simulink model "Model_01_work_2017"  (R2017a)
settings: Solver=VariableStepAuto  StartTime=0.0  StopTime=96  RelTol=1e-3
settings Model: Creator=alexandr.lanin  LastModifiedBy=alexandr.lanin

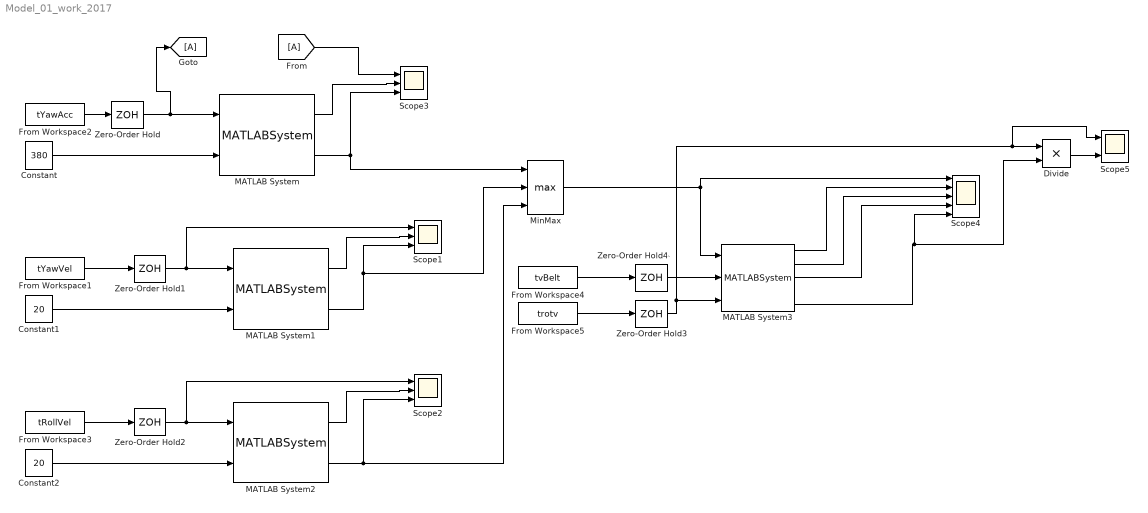
== system Model_01_work_2017 ==
  note: `
  Constant : Constant  Value=380
  Constant1 : Constant  Value=20
  Constant2 : Constant  Value=20
  Divide : Product  Inputs=**
  From Workspace1 : FromWorkspace  VariableName=tYawVel  SampleTime=0
  From Workspace2 : FromWorkspace  VariableName=tYawAcc  SampleTime=0
  From Workspace3 : FromWorkspace  VariableName=tRollVel  SampleTime=0
  From Workspace4 : FromWorkspace  VariableName=tvBelt  SampleTime=0
  From Workspace5 : FromWorkspace  VariableName=trotv  SampleTime=0
  MATLAB System : MATLABSystem  System=WolchSimCode  kMul=100  SimulateUsing=Code generation
      mask Type: WolchSimCode
      mask Display:
      | disp('WolchSimCode');
      | port_label('input',1,'u');
      | port_label('input',2,'norm');
      | port_label('output',1,'Y');
      | port_label('output',2,'Ynorm');
  MATLAB System1 : MATLABSystem  System=WolchSimCode  kMul=100  SimulateUsing=Code generation
      mask Type: WolchSimCode
      mask Display:
      | disp('WolchSimCode');
      | port_label('input',1,'u');
      | port_label('input',2,'norm');
      | port_label('output',1,'Y');
      | port_label('output',2,'Ynorm');
  MATLAB System2 : MATLABSystem  System=WolchSimCode  kMul=100  SimulateUsing=Code generation
      mask Type: WolchSimCode
      mask Display:
      | disp('WolchSimCode');
      | port_label('input',1,'u');
      | port_label('input',2,'norm');
      | port_label('output',1,'Y');
      | port_label('output',2,'Ynorm');
  MATLAB System3 : MATLABSystem  System=ModulSigmoid  Rwheel=17*0.0254  Transfer=3  Kreset=0.6  sd=6  sdsn=0.25  betta=0.6  sm_bet=0.3  alfa=1.0  sm_alfa=0.3  kStd=4  alfaExp=0.75  SimulateUsing=Code generation
      mask Type: ModulSigmoid
      mask Display:
      | disp('ModulSigmoid');
      | port_label('input',1,'signal');
      | port_label('input',2,'vBelt');
      | port_label('input',3,'rotv');
      | port_label('output',1,'y');
      | port_label('output',2,'k');
      | port_label('output',3,'v');
      | port_label('output',4,'ye');
      | port_label('output',5,'yinver');
  MinMax : MinMax  Function=max  Inputs=3
  Scope1 : Scope  NumInputPorts=3
  Scope2 : Scope  NumInputPorts=3
  Scope3 : Scope  NumInputPorts=3
  Scope4 : Scope  NumInputPorts=5
  Scope5 : Scope  NumInputPorts=2
  Zero-Order Hold{,1..4} (5 alike) : ZeroOrderHold  SampleTime=0.01
  wires:
  From Workspace2/1 -> Zero-Order Hold/1
  Zero-Order Hold/1 -> [A], MATLAB System/1
  MATLAB System/1 -> Scope3/2
  MATLAB System/2 -> MinMax/1, Scope3/3
  Constant/1 -> MATLAB System/2
  MATLAB System1/2 -> Scope1/3, MinMax/2
  Constant1/1 -> MATLAB System1/2
  MATLAB System1/1 -> Scope1/2
  From Workspace1/1 -> Zero-Order Hold1/1
  Zero-Order Hold1/1 -> Scope1/1, MATLAB System1/1
  MATLAB System2/1 -> Scope2/2
  From Workspace3/1 -> Zero-Order Hold2/1
  MATLAB System2/2 -> MinMax/3, Scope2/3
  Zero-Order Hold2/1 -> Scope2/1, MATLAB System2/1
  Constant2/1 -> MATLAB System2/2
  [A] -> Scope3/1
  MinMax/1 -> MATLAB System3/1, Scope4/1
  MATLAB System3/1 -> Scope4/2
  From Workspace4/1 -> Zero-Order Hold4/1
  From Workspace5/1 -> Zero-Order Hold3/1
  MATLAB System3/2 -> Scope4/3
  MATLAB System3/3 -> Scope4/4
  Zero-Order Hold4/1 -> MATLAB System3/2
  Zero-Order Hold3/1 -> Scope5/1, Divide/1, MATLAB System3/3
  MATLAB System3/5 -> Divide/2, Scope4/5
  Divide/1 -> Scope5/2
